simulink model "battery_2rc"  (R2022b)
settings: Solver=VariableStepAuto  StartTime=0.0  StopTime=10.0  RelTol=1e-3
undefined symbols (not defined in the file): Battery, I_cc, I_gain, P_gain, R_bleed, T_volt, V_top
libraries: fl_lib x28, nesl_utility x18, simulink x3, batteryecm_lib x3, ee_lib x3, slpidlib x1
(part 1 of 2)
settings Model: Creator=harry  LastModifiedBy=harry

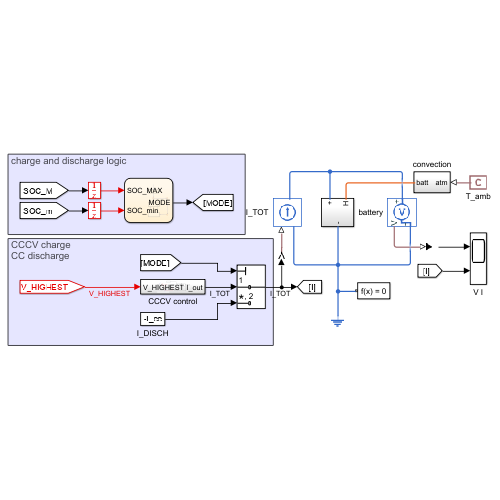
[thumbnail: Simulink's stored preview of the top-level diagram]
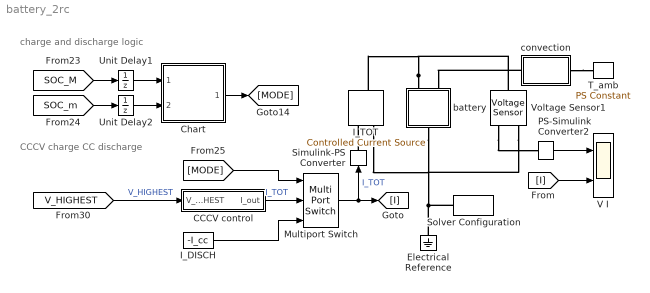
== system battery_2rc ==
  note: charge and discharge logic
  note: CCCV charge
      | CC discharge
  CCCV control : Subsystem
  Chart : Stateflow chart  TreatAsAtomicUnit=on
  Electrical Reference : fl_lib/Electrical/Electrical Elements/Electrical Reference
  I_DISCH : Constant  Value=-I_cc
  I_TOT : fl_lib/Electrical/Electrical Sources/Controlled Current Source
  Multiport Switch : MultiPortSwitch  DataPortOrder=Specify indices  DataPortIndices={1,2}  DiagnosticForDefault=None  SaturateOnIntegerOverflow=off  InputSameDT=off
  PS-Simulink Converter2 : nesl_utility/PS-Simulink Converter  PhysicalDomain=network_engine_domain  SubClassName=ps_output  LeftPortType=input  RightPortType=output  PseudoPeriodic=off  Frequencies=[]  VectorFormat=1-D array  Unit=1  AffineConversion=off
  Simulink-PS Converter : nesl_utility/Simulink-PS Converter  PhysicalDomain=network_engine_domain  SubClassName=ps_input  LeftPortType=input  RightPortType=output  PseudoPeriodic=off  Frequencies=[]  NoiseDistribution=none  NoiseParameters=[]  Unit=1  AffineConversion=off  FilteringAndDerivatives=provide  SimscapeFilterOrder=1  InputFilterTimeConstant=0.001  UdotUserProvided=0
  Solver Configuration : nesl_utility/Solver Configuration  PhysicalDomain=network_engine_domain  SubClassName=solver  LeftPortType=input  RightPortType=generic  Tones=[]  Harmonics=[]  SimulateNoise=off  Profile=off  UseLocalSampling=off  EnableSwitchedLinearOptims=on  FrequencyDomain=off  UseCCode=off  RelTol=0.001  AbsTol=1e-06  MinStep=1e-09  ToWorkspace=off  RevertToSquareIcSolve=off  NumHomotopyIterations=100  PhasorMode=off  PhasorModeNumHarmonics=1  ConsistencySolver=NEWTON_FTOL  IndexReductionMethod=DerivativeReplacement  DoDC=off  ResidualTolerance=1e-09  ConsistencyTolSource=GLOBAL  ConsistencyAbsTol=0.001  ConsistencyRelTol=0.001  ConsistencyTolFactor=0.001  UseLocalSolver=on  LocalSolverChoice=NE_BACKWARD_EULER_ADVANCER  ResolveIndetEquations=on  FunctionEvalNumThread=1  LocalSolverSampleTime=1  DoFixedCost=on  MaxNonlinIter=3  MaxModeIter=2  ComputeImpulses=off  ImpulseIterations=2  LinearAlgebra=Sparse  LinearAlgebraNumThread=0  EquationFormulation=NE_TIME_EF  DelaysMemoryBudget=1024  AutomaticFiltering=on  FilteringTimeConstant=0.001  PartitionStorageMethod=AS_NEEDED  PartitionMemoryBudget=1024  PartitionMethod=FAST
  T_amb : fl_lib/Physical Signals/Sources/PS Constant  constant=20+273
  Unit Delay1 : UnitDelay  InitialCondition=1  SampleTime=-1  HasFrameUpgradeWarning=on
  Unit Delay2 : UnitDelay  InitialCondition=1  SampleTime=-1  HasFrameUpgradeWarning=on
  V I : Scope  NumInputPorts=2
  Voltage Sensor1 : fl_lib/Electrical/Electrical Sensors/Voltage Sensor
  battery : Subsystem
  convection : Subsystem
  wires:
  I_DISCH/1 -> Multiport Switch/3
  Unit Delay2/1 -> Chart/2(SOC_min)
  [MODE] -> Multiport Switch/1
  [SOC_M] -> Unit Delay1/1
  Unit Delay1/1 -> Chart/1(SOC_MAX)
  [SOC_m] -> Unit Delay2/1
  [V_HIGHEST] -> CCCV control/1(V_HIGHEST)  "V_HIGHEST"
  CCCV control/1(I_out) -> Multiport Switch/2  "I_TOT"
  Chart/1(MODE) -> [MODE]
  PS-Simulink Converter2/1 -> V I/1
  Multiport Switch/1 -> Simulink-PS Converter/1, [I]  "I_TOT"
  [I] -> V I/2
  connections:
  battery/LConn1 -- Voltage Sensor1/LConn1 -- I_TOT/LConn1
  Solver Configuration/RConn1 -- Electrical Reference/LConn1 -- I_TOT/RConn2 -- Voltage Sensor1/RConn2 -- battery/RConn1
  convection/LConn1 -- battery/LConn2
  convection/RConn1 -- T_amb/RConn1
  Voltage Sensor1/RConn1 -- PS-Simulink Converter2/LConn1
  Simulink-PS Converter/RConn1 -- I_TOT/RConn1

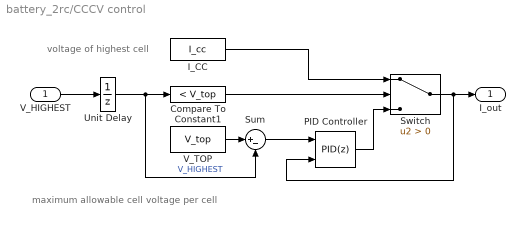
== system battery_2rc/CCCV control ==
  note: maximum allowable cell voltage per cell
  note: voltage of highest cell
  V_HIGHEST : Inport
  Compare To Constant1 : simulink/Logic and Bit Operations/Compare To Constant  relop=<  const=V_top  OutDataTypeStr=boolean
  I_CC : Constant  Value=I_cc
  PID Controller : slpidlib/PID Controller  Controller=PID  Form=Parallel  TimeDomain=Discrete-time  UseExternalTs=off  SampleTime=1  IntegratorMethod=Forward Euler  FilterMethod=Forward Euler  ControllerParametersSource=internal  P=P_gain  I=I_gain  UseKiTs=off  D=0  N=100  UseFilter=on  TunerSelectOption=Transfer Function Based (PID Tuner App)  InitialConditionSource=internal  InitialConditionForIntegrator=10  InitialConditionForFilter=0  DifferentiatorICPrevScaledInput=0  ExternalReset=none  TrackingMode=on  Kt=1  LimitOutput=on  SatLimitsSource=internal  UpperSaturationLimit=Inf  LowerSaturationLimit=0  LinearizeAsGain=on  AntiWindupMode=clamping  Kb=1  LimitIntegrator=off  UpperIntegratorSaturationLimit=inf  LowerIntegratorSaturationLimit=-inf  POutMin=[]  POutMax=[]  IOutMin=[]  IOutMax=[]  DOutMin=[]  DOutMax=[]  NOutMin=[]  NOutMax=[]  SumOutMin=[]  SumOutMax=[]  SaturationOutMin=[]  SaturationOutMax=[]  PParamMin=[]  PParamMax=[]  IParamMin=[]  IParamMax=[]  DParamMin=[]  DParamMax=[]  NParamMin=[]  NParamMax=[]  KbParamMin=[]  KbParamMax=[]  KtParamMin=[]  KtParamMax=[]  KbOutMin=[]  KbOutMax=[]  KtOutMin=[]  KtOutMax=[]  IntegratorOutMin=[]  IntegratorOutMax=[]  FilterOutMin=[]  FilterOutMax=[]  SumI1OutMin=[]  SumI1OutMax=[]  SumI2OutMin=[]  SumI2OutMax=[]  SumI3OutMin=[]  SumI3OutMax=[]  SumI4OutMin=[]  SumI4OutMax=[]  SumDOutMin=[]  SumDOutMax=[]  DifferentiatorOutMin=[]  DifferentiatorOutMax=[]  FilterDiffOutCoefMin=[]  FilterDiffOutCoefMax=[]  ReciprocalOutMin=[]  ReciprocalOutMax=[]  SumDenOutMin=[]  SumDenOutMax=[]  SumNumOutMin=[]  SumNumOutMax=[]  DivideOutMin=[]  DivideOutMax=[]  UdiffTsProdOutMin=[]  UdiffTsProdOutMax=[]  NTsProdOutMin=[]  NTsProdOutMax=[]  UintegralTsProdOutMin=[]  UintegralTsProdOutMax=[]  UngainTsProdOutMin=[]  UngainTsProdOutMax=[]  ClampingZeroOutDataTypeStr=Inherit: Inherit via back propagation  ClampingZeroOutMin=[]  ClampingZeroOutMax=[]  FilterDenConstantOutDataTypeStr=Inherit: Inherit via back propagation  FilterDenConstantOutMin=[]  FilterDenConstantOutMax=[]  PCopyOutDataTypeStr=Inherit: Inherit via back propagation  PCopyOutMin=[]  PCopyOutMax=[]  NCopyOutDataTypeStr=Inherit: Inherit via back propagation  NCopyOutMin=[]  NCopyOutMax=[]  IntegratorContinuousStateAttributes=''  IntegratorStateMustResolveToSignalObject=off  IntegratorRTWStateStorageClass=Auto  FilterContinuousStateAttributes=''  FilterStateMustResolveToSignalObject=off  FilterRTWStateStorageClass=Auto  ParallelPVariant=InternalParameters  IdealPVariant=Disabled  IVariant=InternalParameters  DVariant=InternalParameters  IntegratorVariant=Discrete  SatVariant=Enabled  AWVariant=DiscClampingParallel  PCopyVariant=Disabled  TRVariant=Enabled  FdbkBlocksVariant=Forward  IdealPFdbkVariant=Disabled  SatFdbkVariant=Disabled  DerivativeFilterVariant=ForwardEulerFilter  NVariant=InternalParameters  NCopyVariant=Disabled  FilterICVariant=InternalICsFilter  IntegratorICVariant=InternalICs  ExternalResetVariant=Disabled  TRSumVariant=TrackingMode  SumFdbkVariant=Disabled  SumVariant=Sum_PID  TsampFilterVariant=InternalTs  TsampNgainVariant=Passthrough  TsampIntegralVariant=Passthrough  ExternalSaturationOutDataTypeStr=Inherit: Same as second input
  Sum : Sum  Inputs=|+-
  Switch : Switch  Criteria=u2 > Threshold  SaturateOnIntegerOverflow=off  InputSameDT=off
  Unit Delay : UnitDelay  SampleTime=-1  HasFrameUpgradeWarning=on
  V_TOP : Constant  Value=V_top
  I_out : Outport
  wires:
  Switch/1 -> I_out/1, PID Controller/2
  Unit Delay/1 -> Sum/2, Compare To Constant1/1  "V_HIGHEST"
  PID Controller/1 -> Switch/3
  Sum/1 -> PID Controller/1
  V_TOP/1 -> Sum/1
  I_CC/1 -> Switch/1
  V_HIGHEST/1 -> Unit Delay/1
  Compare To Constant1/1 -> Switch/2

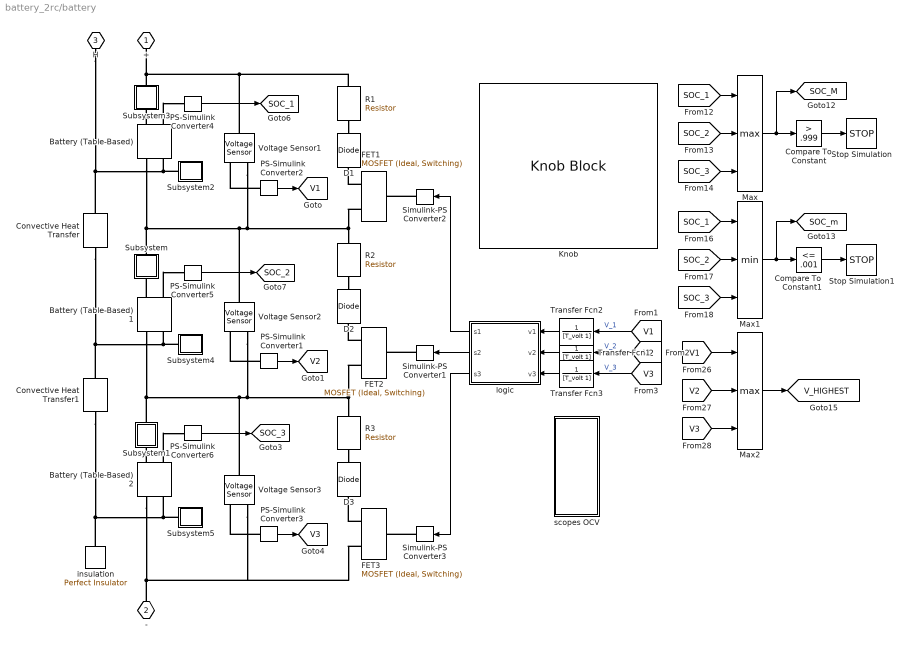
== system battery_2rc/battery ==
  Battery (Table-Based) : batteryecm_lib/Battery (Table-Based)  SOC_vec=Battery(1).SOC_LUT  T_dependence=simscape.enum.tablebattery.temperature_dependence.yes  prm_dir=simscape.enum.tablebattery.prm_dir.noCurrentDirectionality  T_vec=Battery(1).Temperature_LUT K  V0_mat=Battery(1).Em_LUT V  V0_vec=[3.1, 3.27, 3.31, 3.5] V  V_range=[0, inf] V  R0_mat=Battery(1).R0_LUT Ohm  R0_vec=[.015, .017, .012, .013] Ohm  R0_dis_mat=[.0117, .0085, .009; .011, .0085, .009; .0114, .0087, .0092; .0107, .0082, .0088; .0107, .0083, .0091; .0113, .0085, .0089; .0116, .0085, .0089] Ohm  R0_dis_vec=[.0085, .0085, .0087, .0082, .0083, .0085, .0085] Ohm  R0_ch_mat=[.0117, .0085, .009; .011, .0085, .009; .0114, .0087, .0092; .0107, .0082, .0088; .0107, .0083, .0091; .0113, .0085, .0089; .0116, .0085, .0089] Ohm  R0_ch_vec=[.0085, .0085, .0087, .0082, .0083, .0085, .0085] Ohm  AH=Battery(1).Capacity_LUT hr*A  prm_leak=simscape.enum.tablebattery.prm_leak.disabled  Rleak_vec=[8000, 7000, 6000] Ohm  Rleak=7e3 Ohm  extrapolation_option=simscape.enum.extrapolation.linear  SOC_port=simscape.enum.tablebattery.enable.yes  prm_dyn=simscape.enum.tablebattery.prm_dyn.rc3  R1_mat=Battery(1).R1_LUT Ohm  R1_vec=[.076, .022, .007, .043] Ohm  tau1_mat=Battery(1).t1_LUT s  tau1_vec=[148, 110, 27, 22] s  R2_mat=Battery(1).R2_LUT Ohm  R2_vec=[.382, .006, .007, .956] Ohm  tau2_mat=Battery(1).t2_LUT s  tau2_vec=[44, 24, 14, 13419] s  R3_mat=Battery(1).R3_LUT Ohm  R3_vec=[.382, .006, .007, .956] Ohm  tau3_mat=Battery(1).t3_LUT s  tau3_vec=[44, 24, 14, 13419] s  R4_mat=[.014, .382, .407; .028, .006, .007; .014, .007, .006; .333, .956, .912] Ohm  R4_vec=[.382, .006, .007, .956] Ohm  tau4_mat=[1, 44, 5644; 11, 24, 506; 2, 14, 330; 3310, 13419, 30216] s  tau4_vec=[44, 24, 14, 13419] s  R5_mat=[.014, .382, .407; .028, .006, .007; .014, .007, .006; .333, .956, .912] Ohm  R5_vec=[.382, .006, .007, .956] Ohm  tau5_mat=[1, 44, 5644; 11, 24, 506; 2, 14, 330; 3310, 13419, 30216] s  tau5_vec=[44, 24, 14, 13419] s  prm_fade=simscape.enum.tablebattery.prm_fade.equations  N0=100  dV0=0  dR0=0  dAH=0  dRleak=0  dR1=0  dR2=0  dR3=0  dR4=0  dR5=0  N0vec=[100, 200, 300]  Tfadevec=[298.15, 323.15] K  dV0vec=[0, 0, 0]  dR0vec=[0, 0, 0]  dAHvec=[0, 0, 0]  dRleakvec=[0, 0, 0]  dR1vec=[0, 0, 0]  dR2vec=[0, 0, 0]  dR3vec=[0, 0, 0]  dR4vec=[0, 0, 0]  dR5vec=[0, 0, 0]  dV0mat=[0, 0; 0, 0; 0, 0]  dR0mat=[0, 0; 0, 0; 0, 0]  dAHmat=[0, 0; 0, 0; 0, 0]  dRleakmat=[0, 0; 0, 0; 0, 0]  dR1mat=[0, 0; 0, 0; 0, 0]  dR2mat=[0, 0; 0, 0; 0, 0]  dR3mat=[0, 0; 0, 0; 0, 0]  dR4mat=[0, 0; 0, 0; 0, 0]  dR5mat=[0, 0; 0, 0; 0, 0]  prm_age_modeling=simscape.enum.tablebattery.prm_age_modeling.equation  storage_dt_age_vec=[0] d  storage_T_age_vec=[273] K  prm_age_OCV=simscape.enum.tablebattery.prm_age_OCV.OCV  OCV_age=0.9  SOC_age=0.6  prm_age_resistance=simscape.enum.tablebattery.prm_age.disabled  OCV_scaling_age_resistance=2.2134e6  OCV_offset_age_resistance=1.632e6  temp_exp_age_resistance=0.515833569 V  t_exp_age_resistance=0.75  T_age_vec_resistance=[273.15, 298.15, 323.15] K  dt_age_vec_resistance=[90, 180, 270, 360] d  dR0_age_vec=[0, 0, 0]  t_meas_dR0_age=100 d  dR0_age_mat=[0, 0, 0; 0, 0, 0; 0, 0, 0; 0, 0, 0]  prm_age_capacity=simscape.enum.tablebattery.prm_age.disabled  OCV_scaling_age_capacity=1.5097e07  OCV_offset_age_capacity=8.3625e06  temp_exp_age_capacity=0.6011 V  t_exp_age_capacity=0.75  T_age_vec_capacity=[273.15, 298.15, 323.15] K  dt_age_vec_capacity=[90, 180, 270, 360] d  dAH_age_vec=[0, 0, 0]  t_meas_dAH_age=100 d  dAH_age_mat=[0, 0, 0; 0, 0, 0; 0, 0, 0; 0, 0, 0]  thermal_port=simscape.enum.thermaleffects.model  temperature=Battery(1).T_init K  thermal_mass=Battery(1).cell_Cp_heat * Battery(1).cell_mass J/K  i_specify=off  i_priority=None  i=0 A  i_nominal_specify=off  i_nominal_unit=A  i_nominal_value=1  v_specify=off  v_priority=None  v=0 V  v_nominal_specify=off  v_nominal_unit=V  v_nominal_value=1  stateOfCharge_specify=on  stateOfCharge_priority=High  stateOfCharge=Battery(1).SOC0  stateOfCharge_nominal_specify=off  stateOfCharge_nominal_unit=1  stateOfCharge_nominal_value=1  num_cycles_specify=off  num_cycles_priority=High  num_cycles=0  num_cycles_nominal_specify=off  num_cycles_nominal_unit=1  num_cycles_nominal_value=1  cell_temperature_specify=on  cell_temperature_priority=High  cell_temperature=Battery(1).T_init K  cell_temperature_nominal_specify=off  cell_temperature_nominal_unit=K  cell_temperature_nominal_value=1
  Battery (Table-Based)1 : batteryecm_lib/Battery (Table-Based)  SOC_vec=Battery(2).SOC_LUT  T_dependence=simscape.enum.tablebattery.temperature_dependence.yes  prm_dir=simscape.enum.tablebattery.prm_dir.noCurrentDirectionality  T_vec=Battery(2).Temperature_LUT K  V0_mat=Battery(2).Em_LUT V  V0_vec=[3.1, 3.27, 3.31, 3.5] V  V_range=[0, inf] V  R0_mat=Battery(2).R0_LUT Ohm  R0_vec=[.015, .017, .012, .013] Ohm  R0_dis_mat=[.0117, .0085, .009; .011, .0085, .009; .0114, .0087, .0092; .0107, .0082, .0088; .0107, .0083, .0091; .0113, .0085, .0089; .0116, .0085, .0089] Ohm  R0_dis_vec=[.0085, .0085, .0087, .0082, .0083, .0085, .0085] Ohm  R0_ch_mat=[.0117, .0085, .009; .011, .0085, .009; .0114, .0087, .0092; .0107, .0082, .0088; .0107, .0083, .0091; .0113, .0085, .0089; .0116, .0085, .0089] Ohm  R0_ch_vec=[.0085, .0085, .0087, .0082, .0083, .0085, .0085] Ohm  AH=Battery(2).Capacity_LUT hr*A  prm_leak=1  Rleak_vec=[8000, 7000, 6000] Ohm  Rleak=7e3 Ohm  extrapolation_option=simscape.enum.extrapolation.linear  SOC_port=simscape.enum.tablebattery.enable.yes  prm_dyn=4  R1_mat=Battery(2).R1_LUT Ohm  R1_vec=[.076, .022, .007, .043] Ohm  tau1_mat=Battery(2).t1_LUT s  tau1_vec=[148, 110, 27, 22] s  R2_mat=Battery(2).R2_LUT Ohm  R2_vec=[.382, .006, .007, .956] Ohm  tau2_mat=Battery(2).t2_LUT s  tau2_vec=[44, 24, 14, 13419] s  R3_mat=Battery(2).R3_LUT Ohm  R3_vec=[.382, .006, .007, .956] Ohm  tau3_mat=Battery(2).t3_LUT s  tau3_vec=[44, 24, 14, 13419] s  R4_mat=[.014, .382, .407; .028, .006, .007; .014, .007, .006; .333, .956, .912] Ohm  R4_vec=[.382, .006, .007, .956] Ohm  tau4_mat=[1, 44, 5644; 11, 24, 506; 2, 14, 330; 3310, 13419, 30216] s  tau4_vec=[44, 24, 14, 13419] s  R5_mat=[.014, .382, .407; .028, .006, .007; .014, .007, .006; .333, .956, .912] Ohm  R5_vec=[.382, .006, .007, .956] Ohm  tau5_mat=[1, 44, 5644; 11, 24, 506; 2, 14, 330; 3310, 13419, 30216] s  tau5_vec=[44, 24, 14, 13419] s  prm_fade=simscape.enum.tablebattery.prm_fade.equations  N0=100  dV0=0  dR0=0  dAH=0  dRleak=0  dR1=0  dR2=0  dR3=0  dR4=0  dR5=0  N0vec=[100, 200, 300]  Tfadevec=[298.15, 323.15] K  dV0vec=[0, 0, 0]  dR0vec=[0, 0, 0]  dAHvec=[0, 0, 0]  dRleakvec=[0, 0, 0]  dR1vec=[0, 0, 0]  dR2vec=[0, 0, 0]  dR3vec=[0, 0, 0]  dR4vec=[0, 0, 0]  dR5vec=[0, 0, 0]  dV0mat=[0, 0; 0, 0; 0, 0]  dR0mat=[0, 0; 0, 0; 0, 0]  dAHmat=[0, 0; 0, 0; 0, 0]  dRleakmat=[0, 0; 0, 0; 0, 0]  dR1mat=[0, 0; 0, 0; 0, 0]  dR2mat=[0, 0; 0, 0; 0, 0]  dR3mat=[0, 0; 0, 0; 0, 0]  dR4mat=[0, 0; 0, 0; 0, 0]  dR5mat=[0, 0; 0, 0; 0, 0]  prm_age_modeling=simscape.enum.tablebattery.prm_age_modeling.equation  storage_dt_age_vec=[0] d  storage_T_age_vec=[273] K  prm_age_OCV=simscape.enum.tablebattery.prm_age_OCV.OCV  OCV_age=0.9  SOC_age=0.6  prm_age_resistance=simscape.enum.tablebattery.prm_age.disabled  OCV_scaling_age_resistance=2.2134e6  OCV_offset_age_resistance=1.632e6  temp_exp_age_resistance=0.515833569 V  t_exp_age_resistance=0.75  T_age_vec_resistance=[273.15, 298.15, 323.15] K  dt_age_vec_resistance=[90, 180, 270, 360] d  dR0_age_vec=[0, 0, 0]  t_meas_dR0_age=100 d  dR0_age_mat=[0, 0, 0; 0, 0, 0; 0, 0, 0; 0, 0, 0]  prm_age_capacity=simscape.enum.tablebattery.prm_age.disabled  OCV_scaling_age_capacity=1.5097e07  OCV_offset_age_capacity=8.3625e06  temp_exp_age_capacity=0.6011 V  t_exp_age_capacity=0.75  T_age_vec_capacity=[273.15, 298.15, 323.15] K  dt_age_vec_capacity=[90, 180, 270, 360] d  dAH_age_vec=[0, 0, 0]  t_meas_dAH_age=100 d  dAH_age_mat=[0, 0, 0; 0, 0, 0; 0, 0, 0; 0, 0, 0]  thermal_port=simscape.enum.thermaleffects.model  temperature=Battery(2).T_init K  thermal_mass=Battery(2).cell_Cp_heat * Battery(2).cell_mass J/K  i_specify=off  i_priority=None  i=0 A  i_nominal_specify=off  i_nominal_unit=A  i_nominal_value=1  v_specify=off  v_priority=None  v=0 V  v_nominal_specify=off  v_nominal_unit=V  v_nominal_value=1  stateOfCharge_specify=on  stateOfCharge_priority=High  stateOfCharge=Battery(2).SOC0  stateOfCharge_nominal_specify=off  stateOfCharge_nominal_unit=1  stateOfCharge_nominal_value=1  num_cycles_specify=off  num_cycles_priority=High  num_cycles=0  num_cycles_nominal_specify=off  num_cycles_nominal_unit=1  num_cycles_nominal_value=1  cell_temperature_specify=on  cell_temperature_priority=High  cell_temperature=Battery(2).T_init K  cell_temperature_nominal_specify=off  cell_temperature_nominal_unit=K  cell_temperature_nominal_value=1
  Battery (Table-Based)2 : batteryecm_lib/Battery (Table-Based)  SOC_vec=Battery(3).SOC_LUT  T_dependence=simscape.enum.tablebattery.temperature_dependence.yes  prm_dir=simscape.enum.tablebattery.prm_dir.noCurrentDirectionality  T_vec=Battery(3).Temperature_LUT K  V0_mat=Battery(3).Em_LUT V  V0_vec=[3.1, 3.27, 3.31, 3.5] V  V_range=[0, inf] V  R0_mat=Battery(3).R0_LUT Ohm  R0_vec=[.015, .017, .012, .013] Ohm  R0_dis_mat=[.0117, .0085, .009; .011, .0085, .009; .0114, .0087, .0092; .0107, .0082, .0088; .0107, .0083, .0091; .0113, .0085, .0089; .0116, .0085, .0089] Ohm  R0_dis_vec=[.0085, .0085, .0087, .0082, .0083, .0085, .0085] Ohm  R0_ch_mat=[.0117, .0085, .009; .011, .0085, .009; .0114, .0087, .0092; .0107, .0082, .0088; .0107, .0083, .0091; .0113, .0085, .0089; .0116, .0085, .0089] Ohm  R0_ch_vec=[.0085, .0085, .0087, .0082, .0083, .0085, .0085] Ohm  AH=Battery(3).Capacity_LUT hr*A  prm_leak=1  Rleak_vec=[8000, 7000, 6000] Ohm  Rleak=7e3 Ohm  extrapolation_option=simscape.enum.extrapolation.linear  SOC_port=simscape.enum.tablebattery.enable.yes  prm_dyn=4  R1_mat=Battery(3).R1_LUT Ohm  R1_vec=[.076, .022, .007, .043] Ohm  tau1_mat=Battery(3).t1_LUT s  tau1_vec=[148, 110, 27, 22] s  R2_mat=Battery(3).R2_LUT Ohm  R2_vec=[.382, .006, .007, .956] Ohm  tau2_mat=Battery(3).t2_LUT s  tau2_vec=[44, 24, 14, 13419] s  R3_mat=Battery(3).R3_LUT Ohm  R3_vec=[.382, .006, .007, .956] Ohm  tau3_mat=Battery(3).t3_LUT s  tau3_vec=[44, 24, 14, 13419] s  R4_mat=[.014, .382, .407; .028, .006, .007; .014, .007, .006; .333, .956, .912] Ohm  R4_vec=[.382, .006, .007, .956] Ohm  tau4_mat=[1, 44, 5644; 11, 24, 506; 2, 14, 330; 3310, 13419, 30216] s  tau4_vec=[44, 24, 14, 13419] s  R5_mat=[.014, .382, .407; .028, .006, .007; .014, .007, .006; .333, .956, .912] Ohm  R5_vec=[.382, .006, .007, .956] Ohm  tau5_mat=[1, 44, 5644; 11, 24, 506; 2, 14, 330; 3310, 13419, 30216] s  tau5_vec=[44, 24, 14, 13419] s  prm_fade=simscape.enum.tablebattery.prm_fade.equations  N0=100  dV0=0  dR0=0  dAH=0  dRleak=0  dR1=0  dR2=0  dR3=0  dR4=0  dR5=0  N0vec=[100, 200, 300]  Tfadevec=[298.15, 323.15] K  dV0vec=[0, 0, 0]  dR0vec=[0, 0, 0]  dAHvec=[0, 0, 0]  dRleakvec=[0, 0, 0]  dR1vec=[0, 0, 0]  dR2vec=[0, 0, 0]  dR3vec=[0, 0, 0]  dR4vec=[0, 0, 0]  dR5vec=[0, 0, 0]  dV0mat=[0, 0; 0, 0; 0, 0]  dR0mat=[0, 0; 0, 0; 0, 0]  dAHmat=[0, 0; 0, 0; 0, 0]  dRleakmat=[0, 0; 0, 0; 0, 0]  dR1mat=[0, 0; 0, 0; 0, 0]  dR2mat=[0, 0; 0, 0; 0, 0]  dR3mat=[0, 0; 0, 0; 0, 0]  dR4mat=[0, 0; 0, 0; 0, 0]  dR5mat=[0, 0; 0, 0; 0, 0]  prm_age_modeling=simscape.enum.tablebattery.prm_age_modeling.equation  storage_dt_age_vec=[0] d  storage_T_age_vec=[273] K  prm_age_OCV=simscape.enum.tablebattery.prm_age_OCV.OCV  OCV_age=0.9  SOC_age=0.6  prm_age_resistance=simscape.enum.tablebattery.prm_age.disabled  OCV_scaling_age_resistance=2.2134e6  OCV_offset_age_resistance=1.632e6  temp_exp_age_resistance=0.515833569 V  t_exp_age_resistance=0.75  T_age_vec_resistance=[273.15, 298.15, 323.15] K  dt_age_vec_resistance=[90, 180, 270, 360] d  dR0_age_vec=[0, 0, 0]  t_meas_dR0_age=100 d  dR0_age_mat=[0, 0, 0; 0, 0, 0; 0, 0, 0; 0, 0, 0]  prm_age_capacity=simscape.enum.tablebattery.prm_age.disabled  OCV_scaling_age_capacity=1.5097e07  OCV_offset_age_capacity=8.3625e06  temp_exp_age_capacity=0.6011 V  t_exp_age_capacity=0.75  T_age_vec_capacity=[273.15, 298.15, 323.15] K  dt_age_vec_capacity=[90, 180, 270, 360] d  dAH_age_vec=[0, 0, 0]  t_meas_dAH_age=100 d  dAH_age_mat=[0, 0, 0; 0, 0, 0; 0, 0, 0; 0, 0, 0]  thermal_port=simscape.enum.thermaleffects.model  temperature=Battery(3).T_init K  thermal_mass=Battery(3).cell_Cp_heat * Battery(3).cell_mass J/K  i_specify=off  i_priority=None  i=0 A  i_nominal_specify=off  i_nominal_unit=A  i_nominal_value=1  v_specify=off  v_priority=None  v=0 V  v_nominal_specify=off  v_nominal_unit=V  v_nominal_value=1  stateOfCharge_specify=on  stateOfCharge_priority=High  stateOfCharge=Battery(3).SOC0  stateOfCharge_nominal_specify=off  stateOfCharge_nominal_unit=1  stateOfCharge_nominal_value=1  num_cycles_specify=off  num_cycles_priority=High  num_cycles=0  num_cycles_nominal_specify=off  num_cycles_nominal_unit=1  num_cycles_nominal_value=1  cell_temperature_specify=on  cell_temperature_priority=High  cell_temperature=Battery(3).T_init K  cell_temperature_nominal_specify=off  cell_temperature_nominal_unit=K  cell_temperature_nominal_value=1
  Compare To Constant : simulink/Logic and Bit Operations/Compare To Constant  relop=>  const=.999  OutDataTypeStr=boolean
  Compare To Constant1 : simulink/Logic and Bit Operations/Compare To Constant  relop=<=  const=.001  OutDataTypeStr=boolean
  Convective Heat Transfer : fl_lib/Thermal/Thermal Elements/Convective Heat Transfer  thermal_type=foundation.enum.constant_variable.constant  area=cell_area m^2  heat_tr_coeff=h_conv W/(m^2 * K)  min_heat_tr_coeff=1e-3 W/(K*m^2)  T_specify=off  T_priority=None  T=0 K  T_nominal_specify=off  T_nominal_unit=K  T_nominal_value=1  Q_specify=off  Q_priority=None  Q=0 J/s  Q_nominal_specify=off  Q_nominal_unit=J/s  Q_nominal_value=1
  Convective Heat Transfer1 : fl_lib/Thermal/Thermal Elements/Convective Heat Transfer  thermal_type=foundation.enum.constant_variable.constant  area=cell_area m^2  heat_tr_coeff=h_conv W/(m^2 * K)  min_heat_tr_coeff=1e-3 W/(K*m^2)  T_specify=off  T_priority=None  T=0 K  T_nominal_specify=off  T_nominal_unit=K  T_nominal_value=1  Q_specify=off  Q_priority=None  Q=0 J/s  Q_nominal_specify=off  Q_nominal_unit=J/s  Q_nominal_value=1
  D1 : fl_lib/Electrical/Electrical Elements/Diode  Vf=0.6 V  Ron=0.3 Ohm  Goff=1e-8 1/Ohm  i_specify=off  i_priority=None  i=0 A  i_nominal_specify=off  i_nominal_unit=A  i_nominal_value=1  v_specify=off  v_priority=None  v=0 V  v_nominal_specify=off  v_nominal_unit=V  v_nominal_value=1
      settings: LogSimulationData=on
  D2 : fl_lib/Electrical/Electrical Elements/Diode  Vf=0.6 V  Ron=0.3 Ohm  Goff=1e-8 1/Ohm  i_specify=off  i_priority=None  i=0 A  i_nominal_specify=off  i_nominal_unit=A  i_nominal_value=1  v_specify=off  v_priority=None  v=0 V  v_nominal_specify=off  v_nominal_unit=V  v_nominal_value=1
      settings: LogSimulationData=on
  D3 : fl_lib/Electrical/Electrical Elements/Diode  Vf=0.6 V  Ron=0.3 Ohm  Goff=1e-8 1/Ohm  i_specify=off  i_priority=None  i=0 A  i_nominal_specify=off  i_nominal_unit=A  i_nominal_value=1  v_specify=off  v_priority=None  v=0 V  v_nominal_specify=off  v_nominal_unit=V  v_nominal_value=1
      settings: LogSimulationData=on
  FET1 : ee_lib/Semiconductors & Converters/MOSFET (Ideal, Switching)  port_option=ee.enum.controlport.ps  Rds=0.01 Ohm  Goff=1e-6 1/Ohm  Vth=0.9 V  diode_param=2  diode_Vf=0.8 V  diode_Ron=0.001 Ohm  diode_Goff=1e-5 1/Ohm  diode_C=5e-8 F  diode_iRM=-235 A  diode_iF=300 A  diode_idot=-50 A/us  diode_trr_param=1  diode_trr_factor=3  diode_trr=15 us  diode_Qrr=1.5e+3 s*uA  ids_specify=off  ids_priority=None  ids=0 A  ids_nominal_specify=off  ids_nominal_unit=A  ids_nominal_value=1  vds_specify=off  vds_priority=None  vds=0 V  vds_nominal_specify=off  vds_nominal_unit=V  vds_nominal_value=1  vgs_specify=off  vgs_priority=None  vgs=0 V  vgs_nominal_specify=off  vgs_nominal_unit=V  vgs_nominal_value=1  thermal_loss_option=ee.enum.converters.thermalLossOption.constantvalues  Von_data=[0, 1.8, 3.2, 6, 10, 16; 0, 2, 5.5, 9.5, 15, 25] V  Tj=[298.15, 448.15] K  Iout_data=[0, 20, 40, 60, 80, 100] A  Eon_data=[0, 55.04, 124.57, 235.53, 362.12; 0, 71.25, 161.25, 304.88, 468.75] * 1e-6 J  Eoff_data=[0, 18, 30, 56.1, 76.5; 0, 22.5, 37.5, 70.13, 95.63] * 1e-6 J  Tj_loss=[298.15, 448.15] K  Iout_data_loss=[0, 10, 20, 30, 40] A  Eon_scalar=22.86e-3 J  Eoff_scalar=17.14e-3 J  Voff=300 V  Iout_scalar=600 A  diodeModelType=ee.enum.converters.diodeModelType.pwl  diodeTableType=ee.enum.diode.tableType.IfMat  diode_IfMat=[.07, .12, .19, 1.75, 4.24, 7.32, 11.2; .16, .3, .72, 2.14, 4.02, 6.35, 9.12] A  diode_VfMat=[.9, 1.15, 1.25, 1.5, 1.75, 2.17, 2.6, 2.85; .58, .68, .75, 1.1, 1.38, 1.77, 2.27, 2.7] V  diode_TjVec=[25, 125] degC  diode_VfVec=[.5, .7, .9, 1.3, 1.7, 2.1, 2.5] V  diode_IfVec=[.1, .2, .5, 1, 2, 4, 7, 10] A  diode_Vr=-600 V  diode_Ls=150 nH  diode_Erec=0.03 J  thermal_network_parameterization=ee.enum.thermalNetworkTopology.external  Rth=[.03, .2] K/W  Rth_Cauer=[.03, .1, .2] K/W  Rth_Foster=[.03, .2] K/W  thermal_mass_parameterization=ee.enum.thermalNetwork.timeconstant  thermal_mass=[3, 25] J/K  thermal_mass_Cauer=[3, 10, 25] J/K  thermal_mass_Foster=[33, 50] J/K  thermal_time_constant=[.1, 5] s  thermal_time_constant_Cauer=[.1, 1, 5] s  thermal_time_constant_Foster=[1, 10] s  thermal_mass_initial_temperatures=[25, 25] degC  thermal_mass_initial_temperatures_Cauer=[25, 25, 25] degC  junction_thermal_mass=0.1 J/K  Tvec_initial_Foster=[25, 25, 25, 25] degC  no_thermal_network=0  junction_temperature_specify=off  junction_temperature_priority=None  junction_temperature=25 degC  junction_temperature_nominal_specify=off  junction_temperature_nominal_unit=degC  junction_temperature_nominal_value=1  Qj_specify=off  Qj_priority=None  Qj=0 W  Qj_nominal_specify=off  Qj_nominal_unit=W  Qj_nominal_value=1
  FET2 : ee_lib/Semiconductors & Converters/MOSFET (Ideal, Switching)  port_option=ee.enum.controlport.ps  Rds=0.01 Ohm  Goff=1e-6 1/Ohm  Vth=0.9 V  diode_param=2  diode_Vf=0.8 V  diode_Ron=0.001 Ohm  diode_Goff=1e-5 1/Ohm  diode_C=5e-8 F  diode_iRM=-235 A  diode_iF=300 A  diode_idot=-50 A/us  diode_trr_param=1  diode_trr_factor=3  diode_trr=15 us  diode_Qrr=1.5e+3 s*uA  ids_specify=off  ids_priority=None  ids=0 A  ids_nominal_specify=off  ids_nominal_unit=A  ids_nominal_value=1  vds_specify=off  vds_priority=None  vds=0 V  vds_nominal_specify=off  vds_nominal_unit=V  vds_nominal_value=1  vgs_specify=off  vgs_priority=None  vgs=0 V  vgs_nominal_specify=off  vgs_nominal_unit=V  vgs_nominal_value=1  thermal_loss_option=ee.enum.converters.thermalLossOption.constantvalues  Von_data=[0, 1.8, 3.2, 6, 10, 16; 0, 2, 5.5, 9.5, 15, 25] V  Tj=[298.15, 448.15] K  Iout_data=[0, 20, 40, 60, 80, 100] A  Eon_data=[0, 55.04, 124.57, 235.53, 362.12; 0, 71.25, 161.25, 304.88, 468.75] * 1e-6 J  Eoff_data=[0, 18, 30, 56.1, 76.5; 0, 22.5, 37.5, 70.13, 95.63] * 1e-6 J  Tj_loss=[298.15, 448.15] K  Iout_data_loss=[0, 10, 20, 30, 40] A  Eon_scalar=22.86e-3 J  Eoff_scalar=17.14e-3 J  Voff=300 V  Iout_scalar=600 A  diodeModelType=ee.enum.converters.diodeModelType.pwl  diodeTableType=ee.enum.diode.tableType.IfMat  diode_IfMat=[.07, .12, .19, 1.75, 4.24, 7.32, 11.2; .16, .3, .72, 2.14, 4.02, 6.35, 9.12] A  diode_VfMat=[.9, 1.15, 1.25, 1.5, 1.75, 2.17, 2.6, 2.85; .58, .68, .75, 1.1, 1.38, 1.77, 2.27, 2.7] V  diode_TjVec=[25, 125] degC  diode_VfVec=[.5, .7, .9, 1.3, 1.7, 2.1, 2.5] V  diode_IfVec=[.1, .2, .5, 1, 2, 4, 7, 10] A  diode_Vr=-600 V  diode_Ls=150 nH  diode_Erec=0.03 J  thermal_network_parameterization=ee.enum.thermalNetworkTopology.external  Rth=[.03, .2] K/W  Rth_Cauer=[.03, .1, .2] K/W  Rth_Foster=[.03, .2] K/W  thermal_mass_parameterization=ee.enum.thermalNetwork.timeconstant  thermal_mass=[3, 25] J/K  thermal_mass_Cauer=[3, 10, 25] J/K  thermal_mass_Foster=[33, 50] J/K  thermal_time_constant=[.1, 5] s  thermal_time_constant_Cauer=[.1, 1, 5] s  thermal_time_constant_Foster=[1, 10] s  thermal_mass_initial_temperatures=[25, 25] degC  thermal_mass_initial_temperatures_Cauer=[25, 25, 25] degC  junction_thermal_mass=0.1 J/K  Tvec_initial_Foster=[25, 25, 25, 25] degC  no_thermal_network=0  junction_temperature_specify=off  junction_temperature_priority=None  junction_temperature=25 degC  junction_temperature_nominal_specify=off  junction_temperature_nominal_unit=degC  junction_temperature_nominal_value=1  Qj_specify=off  Qj_priority=None  Qj=0 W  Qj_nominal_specify=off  Qj_nominal_unit=W  Qj_nominal_value=1
  FET3 : ee_lib/Semiconductors & Converters/MOSFET (Ideal, Switching)  port_option=ee.enum.controlport.ps  Rds=0.01 Ohm  Goff=1e-6 1/Ohm  Vth=0.9 V  diode_param=2  diode_Vf=0.8 V  diode_Ron=0.001 Ohm  diode_Goff=1e-5 1/Ohm  diode_C=5e-8 F  diode_iRM=-235 A  diode_iF=300 A  diode_idot=-50 A/us  diode_trr_param=1  diode_trr_factor=3  diode_trr=15 us  diode_Qrr=1.5e+3 s*uA  ids_specify=off  ids_priority=None  ids=0 A  ids_nominal_specify=off  ids_nominal_unit=A  ids_nominal_value=1  vds_specify=off  vds_priority=None  vds=0 V  vds_nominal_specify=off  vds_nominal_unit=V  vds_nominal_value=1  vgs_specify=off  vgs_priority=None  vgs=0 V  vgs_nominal_specify=off  vgs_nominal_unit=V  vgs_nominal_value=1  thermal_loss_option=ee.enum.converters.thermalLossOption.constantvalues  Von_data=[0, 1.8, 3.2, 6, 10, 16; 0, 2, 5.5, 9.5, 15, 25] V  Tj=[298.15, 448.15] K  Iout_data=[0, 20, 40, 60, 80, 100] A  Eon_data=[0, 55.04, 124.57, 235.53, 362.12; 0, 71.25, 161.25, 304.88, 468.75] * 1e-6 J  Eoff_data=[0, 18, 30, 56.1, 76.5; 0, 22.5, 37.5, 70.13, 95.63] * 1e-6 J  Tj_loss=[298.15, 448.15] K  Iout_data_loss=[0, 10, 20, 30, 40] A  Eon_scalar=22.86e-3 J  Eoff_scalar=17.14e-3 J  Voff=300 V  Iout_scalar=600 A  diodeModelType=ee.enum.converters.diodeModelType.pwl  diodeTableType=ee.enum.diode.tableType.IfMat  diode_IfMat=[.07, .12, .19, 1.75, 4.24, 7.32, 11.2; .16, .3, .72, 2.14, 4.02, 6.35, 9.12] A  diode_VfMat=[.9, 1.15, 1.25, 1.5, 1.75, 2.17, 2.6, 2.85; .58, .68, .75, 1.1, 1.38, 1.77, 2.27, 2.7] V  diode_TjVec=[25, 125] degC  diode_VfVec=[.5, .7, .9, 1.3, 1.7, 2.1, 2.5] V  diode_IfVec=[.1, .2, .5, 1, 2, 4, 7, 10] A  diode_Vr=-600 V  diode_Ls=150 nH  diode_Erec=0.03 J  thermal_network_parameterization=ee.enum.thermalNetworkTopology.external  Rth=[.03, .2] K/W  Rth_Cauer=[.03, .1, .2] K/W  Rth_Foster=[.03, .2] K/W  thermal_mass_parameterization=ee.enum.thermalNetwork.timeconstant  thermal_mass=[3, 25] J/K  thermal_mass_Cauer=[3, 10, 25] J/K  thermal_mass_Foster=[33, 50] J/K  thermal_time_constant=[.1, 5] s  thermal_time_constant_Cauer=[.1, 1, 5] s  thermal_time_constant_Foster=[1, 10] s  thermal_mass_initial_temperatures=[25, 25] degC  thermal_mass_initial_temperatures_Cauer=[25, 25, 25] degC  junction_thermal_mass=0.1 J/K  Tvec_initial_Foster=[25, 25, 25, 25] degC  no_thermal_network=0  junction_temperature_specify=off  junction_temperature_priority=None  junction_temperature=25 degC  junction_temperature_nominal_specify=off  junction_temperature_nominal_unit=degC  junction_temperature_nominal_value=1  Qj_specify=off  Qj_priority=None  Qj=0 W  Qj_nominal_specify=off  Qj_nominal_unit=W  Qj_nominal_value=1
  Knob : KnobBlock  ScaleMin=2  ScaleMax=40  TickInterval=2
  Max : MinMax  Function=max  Inputs=3
  Max1 : MinMax  Inputs=3
  Max2 : MinMax  Function=max  Inputs=3
  PS-Simulink Converter{1..6} (6 alike) : nesl_utility/PS-Simulink Converter  PhysicalDomain=network_engine_domain  SubClassName=ps_output  LeftPortType=input  RightPortType=output  PseudoPeriodic=off  Frequencies=[]  VectorFormat=1-D array  Unit=1  AffineConversion=off
  R1 : fl_lib/Electrical/Electrical Elements/Resistor  R=R_bleed Ohm  i_specify=off  i_priority=None  i=0 A  i_nominal_specify=off  i_nominal_unit=A  i_nominal_value=1  v_specify=off  v_priority=None  v=0 V  v_nominal_specify=off  v_nominal_unit=V  v_nominal_value=1
      settings: LogSimulationData=on
  R2 : fl_lib/Electrical/Electrical Elements/Resistor  R=R_bleed Ohm  i_specify=off  i_priority=None  i=0 A  i_nominal_specify=off  i_nominal_unit=A  i_nominal_value=1  v_specify=off  v_priority=None  v=0 V  v_nominal_specify=off  v_nominal_unit=V  v_nominal_value=1
  R3 : fl_lib/Electrical/Electrical Elements/Resistor  R=R_bleed Ohm  i_specify=off  i_priority=None  i=0 A  i_nominal_specify=off  i_nominal_unit=A  i_nominal_value=1  v_specify=off  v_priority=None  v=0 V  v_nominal_specify=off  v_nominal_unit=V  v_nominal_value=1
  Simulink-PS Converter1 : nesl_utility/Simulink-PS Converter  PhysicalDomain=network_engine_domain  SubClassName=ps_input  LeftPortType=input  RightPortType=output  PseudoPeriodic=off  Frequencies=[]  NoiseDistribution=none  NoiseParameters=[]  Unit=1  AffineConversion=off  FilteringAndDerivatives=zero  SimscapeFilterOrder=1  InputFilterTimeConstant=0.001  UdotUserProvided=1
  Simulink-PS Converter2 : nesl_utility/Simulink-PS Converter  PhysicalDomain=network_engine_domain  SubClassName=ps_input  LeftPortType=input  RightPortType=output  PseudoPeriodic=off  Frequencies=[]  NoiseDistribution=none  NoiseParameters=[]  Unit=1  AffineConversion=off  FilteringAndDerivatives=zero  SimscapeFilterOrder=1  InputFilterTimeConstant=0.001  UdotUserProvided=1
  Simulink-PS Converter3 : nesl_utility/Simulink-PS Converter  PhysicalDomain=network_engine_domain  SubClassName=ps_input  LeftPortType=input  RightPortType=output  PseudoPeriodic=off  Frequencies=[]  NoiseDistribution=none  NoiseParameters=[]  Unit=1  AffineConversion=off  FilteringAndDerivatives=zero  SimscapeFilterOrder=1  InputFilterTimeConstant=0.001  UdotUserProvided=1
  Stop Simulation : Stop
  Stop Simulation1 : Stop
  Subsystem : Subsystem
  Subsystem1 : Subsystem
  Subsystem2 : Subsystem
  Subsystem3 : Subsystem
  Subsystem4 : Subsystem
  Subsystem5 : Subsystem
  Transfer Fcn1 : TransferFcn  Denominator=[T_volt 1]
  Transfer Fcn2 : TransferFcn  Denominator=[T_volt 1]
  Transfer Fcn3 : TransferFcn  Denominator=[T_volt 1]
  Voltage Sensor1 : fl_lib/Electrical/Electrical Sensors/Voltage Sensor
  Voltage Sensor2 : fl_lib/Electrical/Electrical Sensors/Voltage Sensor
  Voltage Sensor3 : fl_lib/Electrical/Electrical Sensors/Voltage Sensor
  insulation : fl_lib/Thermal/Thermal Elements/Perfect Insulator  T_specify=off  T_priority=None  T=0 K  T_nominal_specify=off  T_nominal_unit=K  T_nominal_value=1
  logic : Subsystem  Variant=on  VariantControlMode=label  LabelModeActiveChoice=(default)
  scopes OCV : Subsystem
  + : PMIOPort  Side=Left
  - : PMIOPort  Port=2  Side=Right
  H : PMIOPort  Port=3  Side=Left
  tag scope: SOC_1=global, SOC_2=global, SOC_3=global, SOC_M=global, SOC_m=global, V1=global, V2=global, V3=global, V_HIGHEST=global
  wires:
  PS-Simulink Converter1/1 -> [V2]
  PS-Simulink Converter3/1 -> [V3]
  PS-Simulink Converter2/1 -> [V1]
  logic/1(s1) -> Simulink-PS Converter2/1
  logic/2(s2) -> Simulink-PS Converter1/1
  logic/3(s3) -> Simulink-PS Converter3/1
  Transfer Fcn2/1 -> logic/1(v1)
  Transfer Fcn1/1 -> logic/2(v2)
  Transfer Fcn3/1 -> logic/3(v3)
  PS-Simulink Converter4/1 -> [SOC_1]
  PS-Simulink Converter5/1 -> [SOC_2]
  PS-Simulink Converter6/1 -> [SOC_3]
  [V1] -> Transfer Fcn2/1  "V_1"
  [V2] -> Transfer Fcn1/1  "V_2"
  [V3] -> Transfer Fcn3/1  "V_3"
  Max2/1 -> [V_HIGHEST]
  [V1] -> Max2/1
  [V2] -> Max2/2
  [V3] -> Max2/3
  Compare To Constant1/1 -> Stop Simulation1/1
  Max1/1 -> Compare To Constant1/1, [SOC_m]
  [SOC_3] -> Max1/3
  [SOC_2] -> Max1/2
  [SOC_1] -> Max1/1
  Compare To Constant/1 -> Stop Simulation/1
  Max/1 -> Compare To Constant/1, [SOC_M]
  [SOC_3] -> Max/3
  [SOC_2] -> Max/2
  [SOC_1] -> Max/1
  connections:
  R1/RConn1 -- D1/LConn1
  R2/RConn1 -- D2/LConn1
  R3/RConn1 -- D3/LConn1
  FET1/RConn1 -- D1/RConn1
  Subsystem/LConn1 -- Battery (Table-Based)/RConn1 -- Voltage Sensor2/LConn1 -- Voltage Sensor1/RConn2 -- FET1/RConn2 -- R2/LConn1
  FET2/RConn1 -- D2/RConn1
  FET3/RConn1 -- D3/RConn1
  -/RConn1 -- Battery (Table-Based)2/RConn1 -- FET3/RConn2 -- Voltage Sensor3/RConn2
  Voltage Sensor1/LConn1 -- R1/LConn1 -- Subsystem3/LConn1 -- +/RConn1
  Battery (Table-Based)1/RConn1 -- Subsystem1/LConn1 -- Voltage Sensor3/LConn1 -- Voltage Sensor2/RConn2 -- FET2/RConn2 -- R3/LConn1
  PS-Simulink Converter2/LConn1 -- Voltage Sensor1/RConn1
  PS-Simulink Converter1/LConn1 -- Voltage Sensor2/RConn1
  PS-Simulink Converter3/LConn1 -- Voltage Sensor3/RConn1
  Simulink-PS Converter2/RConn1 -- FET1/LConn1
  Simulink-PS Converter1/RConn1 -- FET2/LConn1
  Simulink-PS Converter3/RConn1 -- FET3/LConn1
  Convective Heat Transfer/LConn1 -- H/RConn1 -- Subsystem2/LConn1 -- Battery (Table-Based)/RConn2
  Convective Heat Transfer/RConn1 -- Subsystem4/LConn1 -- Battery (Table-Based)1/RConn2 -- Convective Heat Transfer1/LConn1
  Convective Heat Transfer1/RConn1 -- insulation/LConn1 -- Battery (Table-Based)2/RConn2 -- Subsystem5/LConn1
  Battery (Table-Based)2/LConn1 -- Subsystem1/RConn1
  Battery (Table-Based)1/LConn1 -- Subsystem/RConn1
  Battery (Table-Based)/LConn1 -- Subsystem3/RConn1
  Battery (Table-Based)/LConn2 -- PS-Simulink Converter4/LConn1
  Battery (Table-Based)2/LConn2 -- PS-Simulink Converter6/LConn1
  Battery (Table-Based)1/LConn2 -- PS-Simulink Converter5/LConn1

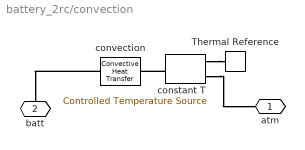
== system battery_2rc/convection ==
  Thermal Reference : fl_lib/Thermal/Thermal Elements/Thermal Reference
  constant T : fl_lib/Thermal/Thermal Sources/Controlled Temperature Source
  convection : fl_lib/Thermal/Thermal Elements/Convective Heat Transfer  thermal_type=foundation.enum.constant_variable.constant  area=cell_area m^2  heat_tr_coeff=h_conv W/(m^2 * K)  min_heat_tr_coeff=1e-3 W/(K*m^2)  T_specify=off  T_priority=None  T=0 K  T_nominal_specify=off  T_nominal_unit=K  T_nominal_value=1  Q_specify=off  Q_priority=None  Q=0 J/s  Q_nominal_specify=off  Q_nominal_unit=J/s  Q_nominal_value=1
  atm : PMIOPort  Side=Right
  batt : PMIOPort  Port=2  Side=Left
  connections:
  convection/LConn1 -- batt/RConn1
  constant T/LConn1 -- convection/RConn1
  constant T/RConn2 -- Thermal Reference/LConn1
  constant T/RConn1 -- atm/RConn1

== system battery_2rc/battery/Subsystem ==
  Subsystem1 : Subsystem
  1 : PMIOPort  Side=Left
  2 : PMIOPort  Port=2  Side=Right
  tag scope: I2=global
  wires:
  Subsystem1/1(3) -> [I2]
  connections:
  Subsystem1/LConn1 -- 1/RConn1
  Subsystem1/RConn1 -- 2/RConn1

== system battery_2rc/battery/Subsystem1 ==
  Subsystem2 : Subsystem
  1 : PMIOPort  Side=Left
  2 : PMIOPort  Port=2  Side=Right
  tag scope: I3=global
  wires:
  Subsystem2/1(3) -> [I3]
  connections:
  Subsystem2/RConn1 -- 2/RConn1
  Subsystem2/LConn1 -- 1/RConn1

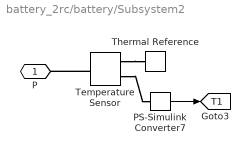
== system battery_2rc/battery/Subsystem2 ==
  PS-Simulink Converter7 : nesl_utility/PS-Simulink Converter  PhysicalDomain=network_engine_domain  SubClassName=ps_output  LeftPortType=input  RightPortType=output  PseudoPeriodic=off  Frequencies=[]  VectorFormat=1-D array  Unit=degC  AffineConversion=on
  Temperature Sensor : fl_lib/Thermal/Thermal Sensors/Temperature Sensor
  Thermal Reference : fl_lib/Thermal/Thermal Elements/Thermal Reference
  P : PMIOPort  Side=Left
  tag scope: T1=global
  wires:
  PS-Simulink Converter7/1 -> [T1]
  connections:
  Temperature Sensor/RConn1 -- Thermal Reference/LConn1
  Temperature Sensor/LConn1 -- P/RConn1
  Temperature Sensor/RConn2 -- PS-Simulink Converter7/LConn1

== system battery_2rc/battery/Subsystem3 ==
  Subsystem : Subsystem
  1 : PMIOPort  Side=Left
  2 : PMIOPort  Port=2  Side=Right
  tag scope: I1=global
  wires:
  Subsystem/1(3) -> [I1]
  connections:
  Subsystem/RConn1 -- 2/RConn1
  Subsystem/LConn1 -- 1/RConn1

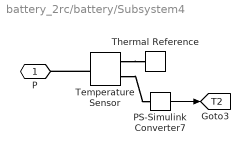
== system battery_2rc/battery/Subsystem4 ==
  PS-Simulink Converter7 : nesl_utility/PS-Simulink Converter  PhysicalDomain=network_engine_domain  SubClassName=ps_output  LeftPortType=input  RightPortType=output  PseudoPeriodic=off  Frequencies=[]  VectorFormat=1-D array  Unit=degC  AffineConversion=on
  Temperature Sensor : fl_lib/Thermal/Thermal Sensors/Temperature Sensor
  Thermal Reference : fl_lib/Thermal/Thermal Elements/Thermal Reference
  P : PMIOPort  Side=Left
  tag scope: T2=global
  wires:
  PS-Simulink Converter7/1 -> [T2]
  connections:
  Temperature Sensor/RConn2 -- PS-Simulink Converter7/LConn1
  Temperature Sensor/LConn1 -- P/RConn1
  Temperature Sensor/RConn1 -- Thermal Reference/LConn1

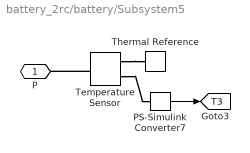
== system battery_2rc/battery/Subsystem5 ==
  PS-Simulink Converter7 : nesl_utility/PS-Simulink Converter  PhysicalDomain=network_engine_domain  SubClassName=ps_output  LeftPortType=input  RightPortType=output  PseudoPeriodic=off  Frequencies=[]  VectorFormat=1-D array  Unit=degC  AffineConversion=on
  Temperature Sensor : fl_lib/Thermal/Thermal Sensors/Temperature Sensor
  Thermal Reference : fl_lib/Thermal/Thermal Elements/Thermal Reference
  P : PMIOPort  Side=Left
  tag scope: T3=global
  wires:
  PS-Simulink Converter7/1 -> [T3]
  connections:
  Temperature Sensor/RConn1 -- Thermal Reference/LConn1
  Temperature Sensor/LConn1 -- P/RConn1
  Temperature Sensor/RConn2 -- PS-Simulink Converter7/LConn1

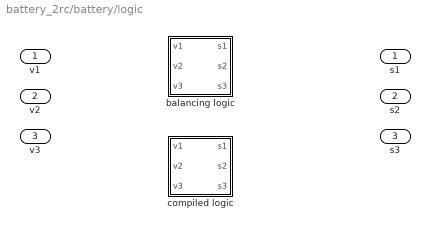
== system battery_2rc/battery/logic ==
  v1 : Inport
  v2 : Inport  Port=2
  v3 : Inport  Port=3
  balancing logic : Stateflow chart  TreatAsAtomicUnit=on  VariantControl=(default)
  compiled logic : Subsystem  VariantControl=Variant
      mask help: Simulink:masks:GenSFuncDesc_MD
      mask Help: eval('feval(''rtwprivate'',''rtwhelpview'',''rtw_sfcn_block'')');
  s1 : Outport  VectorParamsAs1DForOutWhenUnconnected=off
  s2 : Outport  Port=2  VectorParamsAs1DForOutWhenUnconnected=off
  s3 : Outport  Port=3  VectorParamsAs1DForOutWhenUnconnected=off

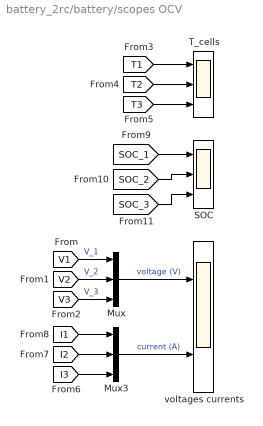
== system battery_2rc/battery/scopes OCV ==
  Mux : Mux  Inputs=3
  Mux3 : Mux  Inputs=3
  SOC : Scope  NumInputPorts=3
  T_cells : Scope  NumInputPorts=3
  voltages currents : Scope  NumInputPorts=2
  wires:
  [I3] -> Mux3/3
  [V1] -> Mux/1  "V_1"
  [V3] -> Mux/3  "V_3"
  Mux/1 -> voltages currents/1  "voltage (V)"
  [V2] -> Mux/2  "V_2"
  [I1] -> Mux3/1
  [I2] -> Mux3/2
  Mux3/1 -> voltages currents/2  "current (A)"
  [SOC_1] -> SOC/1
  [SOC_2] -> SOC/2
  [SOC_3] -> SOC/3
  [T1] -> T_cells/1
  [T2] -> T_cells/2
  [T3] -> T_cells/3

== system battery_2rc/battery/Subsystem/Subsystem1 ==
  Current Sensor : fl_lib/Electrical/Electrical Sensors/Current Sensor
  PS-Simulink Converter4 : nesl_utility/PS-Simulink Converter  PhysicalDomain=network_engine_domain  SubClassName=ps_output  LeftPortType=input  RightPortType=output  PseudoPeriodic=off  Frequencies=[]  VectorFormat=1-D array  Unit=1  AffineConversion=off
  1 : PMIOPort  Side=Left
  2 : PMIOPort  Port=2  Side=Right
  3 : Outport  VectorParamsAs1DForOutWhenUnconnected=off
  wires:
  PS-Simulink Converter4/1 -> 3/1
  connections:
  PS-Simulink Converter4/LConn1 -- Current Sensor/RConn1
  Current Sensor/RConn2 -- 2/RConn1
  Current Sensor/LConn1 -- 1/RConn1

== system battery_2rc/battery/Subsystem1/Subsystem2 ==
  Current Sensor : fl_lib/Electrical/Electrical Sensors/Current Sensor
  PS-Simulink Converter4 : nesl_utility/PS-Simulink Converter  PhysicalDomain=network_engine_domain  SubClassName=ps_output  LeftPortType=input  RightPortType=output  PseudoPeriodic=off  Frequencies=[]  VectorFormat=1-D array  Unit=1  AffineConversion=off
  1 : PMIOPort  Side=Left
  2 : PMIOPort  Port=2  Side=Right
  3 : Outport  VectorParamsAs1DForOutWhenUnconnected=off
  wires:
  PS-Simulink Converter4/1 -> 3/1
  connections:
  PS-Simulink Converter4/LConn1 -- Current Sensor/RConn1
  Current Sensor/RConn2 -- 2/RConn1
  Current Sensor/LConn1 -- 1/RConn1

== system battery_2rc/battery/Subsystem3/Subsystem ==
  Current Sensor : fl_lib/Electrical/Electrical Sensors/Current Sensor
  PS-Simulink Converter4 : nesl_utility/PS-Simulink Converter  PhysicalDomain=network_engine_domain  SubClassName=ps_output  LeftPortType=input  RightPortType=output  PseudoPeriodic=off  Frequencies=[]  VectorFormat=1-D array  Unit=1  AffineConversion=off
  1 : PMIOPort  Side=Left
  2 : PMIOPort  Port=2  Side=Right
  3 : Outport  VectorParamsAs1DForOutWhenUnconnected=off
  wires:
  PS-Simulink Converter4/1 -> 3/1
  connections:
  Current Sensor/LConn1 -- 1/RConn1
  Current Sensor/RConn2 -- 2/RConn1
  PS-Simulink Converter4/LConn1 -- Current Sensor/RConn1

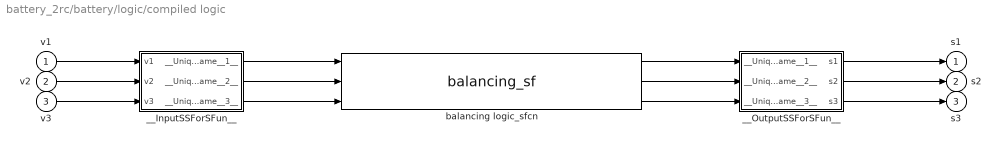
== system battery_2rc/battery/logic/compiled logic ==
  v1 : Inport
  v2 : Inport  Port=2
  v3 : Inport  Port=3
  __InputSSForSFun__ : Subsystem
  __OutputSSForSFun__ : Subsystem
  balancing logic_sfcn : S-Function  FunctionName=balancing_sf  SFunctionModules=""  SFunctionDeploymentMode=off  EnableBusSupport=off  mask{rtw_sf_name=balancing_sf, showVar=off}
      mask prompts: rtw_sf_name "Simulink:masks:GenSFuncName_MP"; showVar "Simulink:masks:GenSFuncShowModuleList_MP"
      mask help: Simulink:masks:GenSFuncDesc_MD
      mask init:
      | displist = '';
      | if ~strcmp(get_param(gcb, 'FunctionName'), rtw_sf_name);
      |   set_param(gcb, 'FunctionName', rtw_sf_name);
      | end
      | % Check if we are generating code
      | rtw_mode = false;
      | if strcmpi(get_param(bdroot(gcb),'SimulationStatus'),'Initializing')
      | 	rtw_mode = strcmpi(get_param(bdroot(gcb),'BuildingRTWCode'),'on') && ...
      | 		~strcmpi(get_param(bdroot(gcb),'TargetStyle'),'SimulationTarget');
      | end
      | if showVar || rtw_mode
      | 	if exist('rtwsfunc') == 2 | exist('rtwsfunc') == 6
      | 		tmplist = rtwsfunc(rtw_sf_name,gcb);
      | 		tmplist = DAStudio.message('Simulink:masks:GenSFuncListOfModules_IC', tmplist);
      | 	elseif showVar
      | 		tmplist1 = DAStudio.message('Simulink:masks:GenSFuncListOfModules_IC', '');
      |         tmplist2 = DAStudio.message('Simulink:masks:GenSFuncNotLicensed_IC');
      |         tmplist = [tmplist1 tmplist2];
      |  	end
      | end
      | if showVar
      |   displist = tmplist;
      | end
      settings: CopyFcn=|
      | if ~strcmp(get_param(gcb,'Linkstatus'),'none') && ...
      | ~strcmp(get_param(gcb,'Linkstatus'),'implicit')
      |   set_param(gcb,'LinkStatus','none');
      | end
      mask Help: eval('feval(''rtwprivate'',''rtwhelpview'',''rtw_sfcn_block'')');
      mask Display:
      | port_label('input',1,'v1');
      | port_label('input',2,'v2');
      | port_label('input',3,'v3');
      | port_label('output',1,'s1');
      | port_label('output',2,'s2');
      | port_label('output',3,'s3');
  s1 : Outport  VectorParamsAs1DForOutWhenUnconnected=off
  s2 : Outport  Port=2  VectorParamsAs1DForOutWhenUnconnected=off
  s3 : Outport  Port=3  VectorParamsAs1DForOutWhenUnconnected=off
  wires:
  __OutputSSForSFun__/3(s3) -> s3/1
  __OutputSSForSFun__/2(s2) -> s2/1
  __OutputSSForSFun__/1(s1) -> s1/1
  balancing logic_sfcn/3 -> __OutputSSForSFun__/3(__UniqueInportName__3__)
  balancing logic_sfcn/2 -> __OutputSSForSFun__/2(__UniqueInportName__2__)
  balancing logic_sfcn/1 -> __OutputSSForSFun__/1(__UniqueInportName__1__)
  __InputSSForSFun__/3(__UniqueOutportName__3__) -> balancing logic_sfcn/3
  __InputSSForSFun__/2(__UniqueOutportName__2__) -> balancing logic_sfcn/2
  __InputSSForSFun__/1(__UniqueOutportName__1__) -> balancing logic_sfcn/1
  v3/1 -> __InputSSForSFun__/3(v3)
  v2/1 -> __InputSSForSFun__/2(v2)
  v1/1 -> __InputSSForSFun__/1(v1)

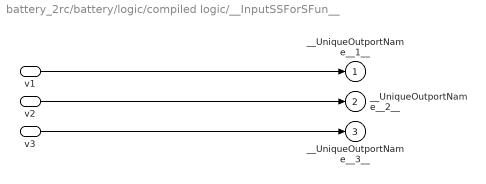
== system battery_2rc/battery/logic/compiled logic/__InputSSForSFun__ ==
  v1 : Inport
  v2 : Inport  Port=2
  v3 : Inport  Port=3
  __UniqueOutportName__1__ : Outport  VectorParamsAs1DForOutWhenUnconnected=off
  __UniqueOutportName__2__ : Outport  Port=2  VectorParamsAs1DForOutWhenUnconnected=off
  __UniqueOutportName__3__ : Outport  Port=3  VectorParamsAs1DForOutWhenUnconnected=off
  wires:
  v3/1 -> __UniqueOutportName__3__/1
  v2/1 -> __UniqueOutportName__2__/1
  v1/1 -> __UniqueOutportName__1__/1

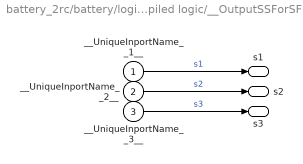
== system battery_2rc/battery/logic/compiled logic/__OutputSSForSFun__ ==
  __UniqueInportName__1__ : Inport
  __UniqueInportName__2__ : Inport  Port=2
  __UniqueInportName__3__ : Inport  Port=3
  s1 : Outport  VectorParamsAs1DForOutWhenUnconnected=off
  s2 : Outport  Port=2  VectorParamsAs1DForOutWhenUnconnected=off
  s3 : Outport  Port=3  VectorParamsAs1DForOutWhenUnconnected=off
  wires:
  __UniqueInportName__3__/1 -> s3/1  "s3"
  __UniqueInportName__2__/1 -> s2/1  "s2"
  __UniqueInportName__1__/1 -> s1/1  "s1"

== stateflow chart battery_2rc/battery/logic/balancing logic ==
  state init
    entry: s1 = 0;
    s2 = 0;
    s3 = 0;
  state finish
    entry: s1 = 0;
    s2 = 0;
    s3 = 0;
  state balancing
    du: sortV = ord(v1,v2,v3);
    state s1_s3
      en: s1 = 1;
      s3 = 1;
      s2 = 0;
      ex: s1 = 0;
      s3 = 0;
      s2 = 0;
    state s1_s2
      en: s1 = 1;
      s2 = 1;
      s3 = 0;
      ex: s1 = 0;
      s2 = 0;
      s3 = 0;
    state s2_s3
      en: s2 = 1;
      s3 = 1;
      s1 = 0;
      ex: s1 = 0;
      s3 = 0;
      s2 = 0;
    (default) -> (junction 382) : {sortV = ord(v1,v2,v3);}
    (junction 382) -> (junction 422) [order 3] : % cell#1 lowest
        | [sortV(1)==1]
    (junction 382) -> (junction 424) [order 2] : % cell#2 lowest
        | [sortV(1)==2]
    (junction 382) -> s1_s2 [order 1] : % cell#3 lowest
        | [sortV(1)==3]
    (junction 422) -> s2_s3
    (junction 424) -> (junction 425)
    (junction 425) -> s1_s3
    s1_s3 -> s2_s3 [order 2] : [sortV(1)==1]
    s1_s2 -> s1_s3 [order 1] : [sortV(1)==2]
    s1_s3 -> s1_s2 [order 1] : [sortV(1)==3]
    s2_s3 -> s1_s3 [order 1] : [sortV(1)==2]
    s1_s2 -> (junction 414) [order 2] : [sortV(1)==1]
    (junction 415) -> s1_s2
    s2_s3 -> (junction 416) [order 2] : [sortV(1)==3]
    (junction 417) -> s2_s3
    (junction 416) -> (junction 415)
    (junction 414) -> (junction 417)
  (default) -> init
  finish -> balancing : [abs(max([v1 v2 v3]) - min([v1 v2 v3])) > deltaV && after(1,sec)]
  balancing -> finish : [abs(max([v1 v2 v3]) - min([v1 v2 v3])) < deltaV]
  init -> balancing : [abs(max([v1 v2 v3]) - min([v1 v2 v3])) > deltaV]
  data: a function_input; b function_input; c function_input; p function_output; v1 input; v2 input; v3 input; s1 output; s2 output; s3 output; deltaV parameter; sortV local
  function p = ord(a,b,c):
    | function p = ord(a,b,c)
    | [~,p] = sort([a,b,c],'ascend');
